simulink model "OFDM_QPSK_Rayleigh_Channel"  (Simulink 7.9)
settings: Solver=FixedStepDiscrete  StartTime=0.0  StopTime=1000  RelTol=1e-3
PreLoadFcn:
  | bitRate = 500000;
  | bitsPerFrame = 200;
  | maxDopplerShift = 200;
  | delayVector = [0:3]*(4e-6);
  | gainVector = [0:3]*(-3);
  | LOSDopplerShift = 100;
  | KFactor = 10;
undefined symbols (not defined in the file or in its folder): figposition, Fs, get, sided, Two
libraries: dspxfrm3 x4, commchan3 x3, commsink2 x2, dspsnks4 x1, dspstat3 x1, commrandsrc2 x1, commdigbbndam3 x1
Description:
  | Multipath Fading Channel
  | 
  | To learn about this model, click <a href="matlab: showdemo multipathfading_demo;">here</a>.
CloseFcn:
  | clear bitRate
  | clear bitsPerFrame
  | clear maxDopplerShift
  | clear delayVector
  | clear gainVector
  | clear LOSDopplerShift
  | clear KFactor
settings Model: Creator=The MathWorks Inc.  LastModifiedBy=leixia  ExtModeAutoUpdateStatusClock=off  BufferReuse=off
settings DataIOCC: LimitDataPoints=off  SaveOutput=off  SignalLogging=off  SaveTime=off  SignalLoggingName=multipathSigsOut
settings OptimizationCC: BooleanDataType=off  InlineInvariantSignals=on  OptimizeBlockIOStorage=off  BufferReuse=off  ExpressionFolding=off  LocalBlockOutputs=off  InitFltsAndDblsToZero=on  BufferReusableBoundary=off
settings DebuggingCC: SaveWithParameterizedLinksMsg=none  CheckExecutionContextPreStartOutputMsg=on  CheckExecutionContextRuntimeOutputMsg=on  SignalResolutionControl=TryResolveAllWithWarning  SolverPrmCheckMsg=none  InheritedTsInSrcMsg=none  MultiTaskDSMMsg=warning  MultiTaskCondExecSysMsg=none  SigSpecEnsureSampleTimeMsg=none  FcnCallInpInsideContextMsg=Use local settings  BusObjectLabelMismatch=none  StrictBusMsg=None
settings HardwareCC: TargetUnknown=on
settings ModelReferenceCC: UpdateModelReferenceTargets=IfOutOfDate
settings RTWCC: IncludeERTFirstTime=on
settings GRTTargetCC: TargetFcnLib=ansi_tfl_tmw.mat  CombineOutputUpdateFcns=off  GRTInterface=on

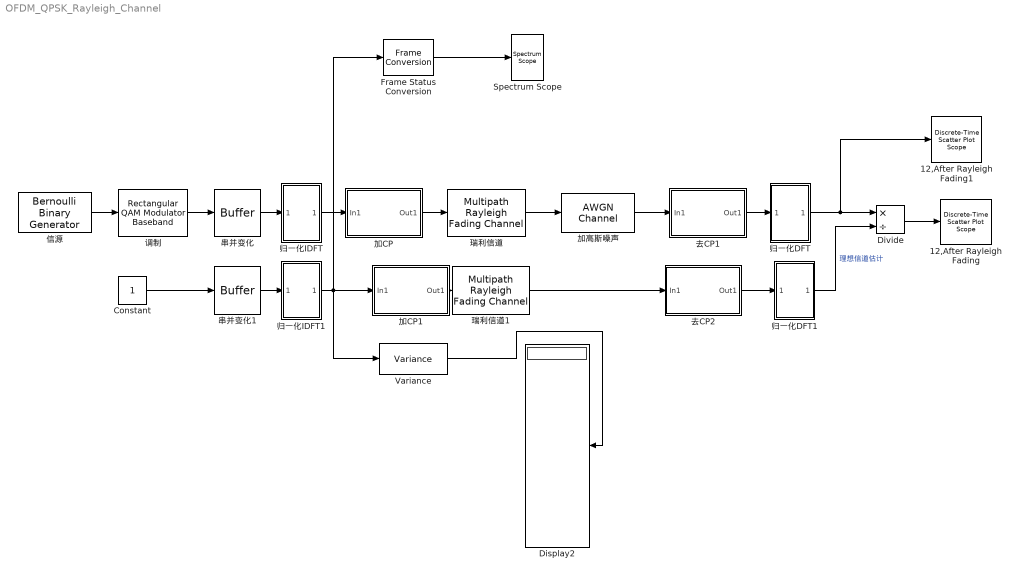
== system OFDM_QPSK_Rayleigh_Channel ==
  12,After Rayleigh Fading : commsink2/Discrete-Time Scatter Plot Scope  Tag=ScatterPlot  sampPerSymb=1  offsetEye=0  numTraces=100  numNewFrames=8  LineMarkers=.  LineColors=b  fading=on  render=on  AxisGrid=on  xMin=-1.2  xMax=1.2  yMin=-1.2  yMax=1.2  inphaseLabel=In-phase Amplitude  quadratureLabel=Quadrature Amplitude  openScopeAtSimStart=off  FrameNumber=off  FigPos=figposition([1 40 25 40])  figTitle=Received signal after Rayleigh fading  numLinesMax=8  block_type_=scatter
  12,After Rayleigh Fading1 : commsink2/Discrete-Time Scatter Plot Scope  Tag=ScatterPlot  sampPerSymb=1  offsetEye=0  numTraces=100  numNewFrames=8  LineMarkers=.  LineColors=b  fading=on  render=on  AxisGrid=on  xMin=-1.2  xMax=1.2  yMin=-1.2  yMax=1.2  inphaseLabel=In-phase Amplitude  quadratureLabel=Quadrature Amplitude  openScopeAtSimStart=off  FrameNumber=off  FigPos=figposition([1 40 25 40])  figTitle=Received signal after Rayleigh fading  numLinesMax=8  block_type_=scatter
  Constant : Constant  VectorParams1D=off  SampleTime=1/500000*2  FramePeriod=256
  Display2 : Display
  Divide : Product  Inputs=*/
  Frame Status Conversion : FrameConversion
  Spectrum Scope : dspsnks4/Spectrum Scope  ScopeProperties=on  Domain=Frequency  HorizSpan=1  UseBuffer=off  BufferSize=272  Overlap=0  TreatMby1Signals=One channel  inpFftLenInherit=off  FFTlength=272  numAvg=1  DisplayProperties=off  AxisGrid=on  Memory=off  FrameNumber=on  AxisLegend=off  AxisZoom=off  OpenScopeAtSimStart=on  OpenScopeImmediately=off  FigPos=get(0,'defaultfigureposition')  AxisProperties=off  XUnits=Hertz  XRange=Two-sided ((-Fs/2...Fs/2])  XDisplay=0  InheritXIncr=on  XIncr=1.0  XLabel=Samples  XLimit=Auto  YUnits=dBW/Hertz  XMax=1  XMin=0  YLabel=Magnitude-squared, dB  LineProperties=off  wintypeSpecScope=Hann  RsSpecScope=50  betaSpecScope=5  winsampSpecScope=Periodic  XAxisParamsVer=6.9  isFrameUpgraded=on
      settings: YMin=-10  YMax=10
  Variance : dspstat3/Variance  run=on  reset_popup=None  InputProcessing=Columns as channels (frame based)  directionMode=Each column  dimension=1  treatSBRowAsCol=on  roiEnable=off  roiType=Rectangles  roiPortion=Entire ROI  roiOutput=Individual statistics for each ROI  roiFlag=off  roundingMode=Floor  overflowMode=off
  串并变化 : Buffer  N=256  TreatMby1Signals=One channel
  串并变化1 : Buffer  N=256  TreatMby1Signals=One channel
  信源 : commrandsrc2/Bernoulli Binary Generator  P=0.5  seed=61  Ts=1/500000  frameBased=on  sampPerFrame=2  orient=off  outDataType=double
  加CP : Subsystem
  加CP1 : Subsystem
  加高斯噪声 : commchan3/AWGN Channel  InputProcessing=Inherited (this choice will be removed - see release notes)  seed=67  noiseMode="Signal to noise ratio  (SNR)"  EbNodB=10  EsNodB=15  SNRdB=200  bitsPerSym=1  Ps=1  Tsym=1e-6  variance=1
  去CP1 : Subsystem
  去CP2 : Subsystem
  归一化DFT : Subsystem
  归一化DFT1 : Subsystem
  归一化IDFT : Subsystem
  归一化IDFT1 : Subsystem
  瑞利信道 : commchan3/Multipath Rayleigh Fading Channel  maxDopplerShift=0.01  spectrumType=Jakes  sigmaGaussian=1/sqrt(2)  coeffRounded=[1 -1.72 0.785]  freqMinMaxRJakes=[0 1]  freqMinMaxAJakes=[0 1]  sigmaGaussian1=1/sqrt(2)  sigmaGaussian2=1/sqrt(2)  centerFreqGaussian1=0.0  centerFreqGaussian2=0.0  gainGaussian1=0.5  gainGaussian2=0.5  coeffBell=9  dopplerSpectrum=doppler.jakes  pathDelays="[ 0    0.0400 ].*1e-4"  avgPathGaindB="[ 0    -3 ]"  normalizePathGains=on  seed=12345  enableProbe=0  openVisAtStart=off  outPathGains=off  outDelay=off
  瑞利信道1 : commchan3/Multipath Rayleigh Fading Channel  maxDopplerShift=0.01  spectrumType=Jakes  sigmaGaussian=1/sqrt(2)  coeffRounded=[1 -1.72 0.785]  freqMinMaxRJakes=[0 1]  freqMinMaxAJakes=[0 1]  sigmaGaussian1=1/sqrt(2)  sigmaGaussian2=1/sqrt(2)  centerFreqGaussian1=0.0  centerFreqGaussian2=0.0  gainGaussian1=0.5  gainGaussian2=0.5  coeffBell=9  dopplerSpectrum=doppler.jakes  pathDelays="[ 0    0.0400 ].*1e-4"  avgPathGaindB="[ 0    -3 ]"  normalizePathGains=on  seed=12345  enableProbe=0  openVisAtStart=off  outPathGains=off  outDelay=off
  调制 : commdigbbndam3/Rectangular QAM Modulator Baseband  M=4  InType=Bit  Enc=Gray  Mapping=[0,1,2,3]  PowType=Average Power  MinDist=2  AvgPow=1  PeakPow=1  Ph=-pi/2  outDtype=double  outWordLen=16  outUDDataType=sfix(16)  outFracLenMode=Best precision  outFracLen=15
  wires:
  调制/1 -> 串并变化/1
  瑞利信道/1 -> 加高斯噪声/1
  加高斯噪声/1 -> 去CP1/1(In1)
  信源/1 -> 调制/1
  加CP/1(Out1) -> 瑞利信道/1
  归一化IDFT/1(Out1) -> 加CP/1(In1)
  串并变化/1 -> 归一化IDFT/1(In1)
  去CP1/1(Out1) -> 归一化DFT/1(In1)
  去CP2/1(Out1) -> 归一化DFT1/1(In1)
  加CP1/1(Out1) -> 瑞利信道1/1
  Constant/1 -> 串并变化1/1
  串并变化1/1 -> 归一化IDFT1/1(In1)
  瑞利信道1/1 -> 去CP2/1(In1)
  归一化DFT/1(Out1) -> Divide/1, 12,After Rayleigh Fading1/1
  归一化DFT1/1(Out1) -> Divide/2  "理想信道估计"
  Divide/1 -> 12,After Rayleigh Fading/1
  Frame Status Conversion/1 -> Spectrum Scope/1
  归一化IDFT1/1(Out1) -> Frame Status Conversion/1, 加CP1/1(In1), Variance/1
  Variance/1 -> Display2/1

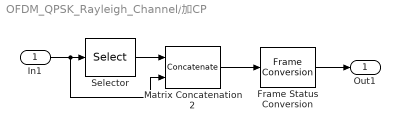
== system OFDM_QPSK_Rayleigh_Channel/加CP ==
  In1 : Inport
  Frame Status Conversion : FrameConversion
  Matrix Concatenation2 : Concatenate
  Selector : Selector  InputPortWidth=256  IndexOptions=Index vector (dialog)  Indices=[256-16+1:1:256]  OutputSizes=1
  Out1 : Outport
  wires:
  Selector/1 -> Matrix Concatenation2/1
  In1/1 -> Matrix Concatenation2/2, Selector/1
  Matrix Concatenation2/1 -> Frame Status Conversion/1
  Frame Status Conversion/1 -> Out1/1

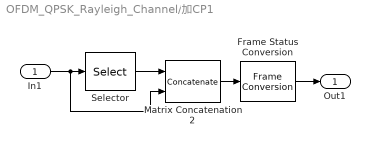
== system OFDM_QPSK_Rayleigh_Channel/加CP1 ==
  In1 : Inport
  Frame Status Conversion : FrameConversion
  Matrix Concatenation2 : Concatenate
  Selector : Selector  InputPortWidth=256  IndexOptions=Index vector (dialog)  Indices=[256-16+1:1:256]  OutputSizes=1
  Out1 : Outport
  wires:
  Frame Status Conversion/1 -> Out1/1
  Matrix Concatenation2/1 -> Frame Status Conversion/1
  In1/1 -> Selector/1, Matrix Concatenation2/2
  Selector/1 -> Matrix Concatenation2/1

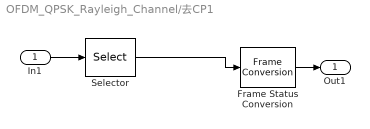
== system OFDM_QPSK_Rayleigh_Channel/去CP1 ==
  In1 : Inport
  Frame Status Conversion : FrameConversion
  Selector : Selector  InputPortWidth=256+16  IndexOptions=Index vector (dialog)  Indices=[16+1:1:256+16]  OutputSizes=1
  Out1 : Outport
  wires:
  Frame Status Conversion/1 -> Out1/1
  In1/1 -> Selector/1
  Selector/1 -> Frame Status Conversion/1

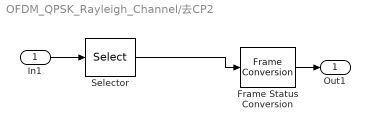
== system OFDM_QPSK_Rayleigh_Channel/去CP2 ==
  In1 : Inport
  Frame Status Conversion : FrameConversion
  Selector : Selector  InputPortWidth=256+16  IndexOptions=Index vector (dialog)  Indices=[16+1:1:256+16]  OutputSizes=1
  Out1 : Outport
  wires:
  Selector/1 -> Frame Status Conversion/1
  In1/1 -> Selector/1
  Frame Status Conversion/1 -> Out1/1

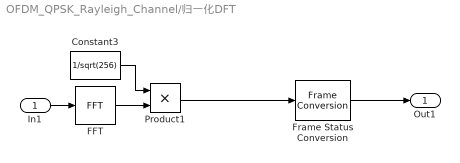
== system OFDM_QPSK_Rayleigh_Channel/归一化DFT ==
  In1 : Inport
  Constant3 : Constant  Value=1/sqrt(256)
  FFT : dspxfrm3/FFT  CompMethod=Table lookup  TableOpt=NEW  TableOptActive=Speed  BitRevOrder=off  InheritFFTLength=on  FFTLength=64  RowConvenienceOn=on  FFTImplementation=Auto  SkipNorm=off  firstCoeffDataTypeStr=Inherit: Same word length as input  firstCoeffLastDataTypeStr=Inherit: Same word length as input  outputMin=[]  outputMax=[]  roundingMode=Floor  overflowMode=off
  Frame Status Conversion : FrameConversion
  Product1 : Product  SaturateOnIntegerOverflow=on  InputSameDT=on  OutDataTypeStr=Inherit: Same as first input
  Out1 : Outport
  wires:
  In1/1 -> FFT/1
  Product1/1 -> Frame Status Conversion/1
  FFT/1 -> Product1/2
  Constant3/1 -> Product1/1
  Frame Status Conversion/1 -> Out1/1

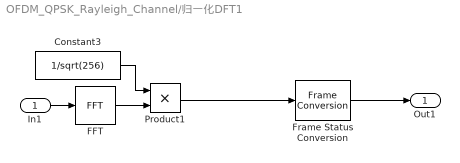
== system OFDM_QPSK_Rayleigh_Channel/归一化DFT1 ==
  In1 : Inport
  Constant3 : Constant  Value=1/sqrt(256)
  FFT : dspxfrm3/FFT  CompMethod=Table lookup  TableOpt=NEW  TableOptActive=Speed  BitRevOrder=off  InheritFFTLength=on  FFTLength=64  RowConvenienceOn=on  FFTImplementation=Auto  SkipNorm=off  firstCoeffDataTypeStr=Inherit: Same word length as input  firstCoeffLastDataTypeStr=Inherit: Same word length as input  outputMin=[]  outputMax=[]  roundingMode=Floor  overflowMode=off
  Frame Status Conversion : FrameConversion
  Product1 : Product  SaturateOnIntegerOverflow=on  InputSameDT=on  OutDataTypeStr=Inherit: Same as first input
  Out1 : Outport
  wires:
  Frame Status Conversion/1 -> Out1/1
  Constant3/1 -> Product1/1
  FFT/1 -> Product1/2
  Product1/1 -> Frame Status Conversion/1
  In1/1 -> FFT/1

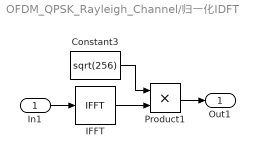
== system OFDM_QPSK_Rayleigh_Channel/归一化IDFT ==
  In1 : Inport
  Constant3 : Constant  Value=sqrt(256)
  IFFT : dspxfrm3/IFFT  CompMethod=Table lookup  TableOpt=NEW  TableOptActive=Speed  BitRevOrder=off  cs_in=off  SkipNorm=on  InheritFFTLength=on  FFTLength=64  mode=Complex  outSamplingMode=Sample based  RowConvenienceOn=on  FFTImplementation=Auto  firstCoeffDataTypeStr=Inherit: Same word length as input  firstCoeffLastDataTypeStr=Inherit: Same word length as input  outputMin=[]  outputMax=[]  roundingMode=Floor  overflowMode=off
  Product1 : Product  SaturateOnIntegerOverflow=on  InputSameDT=on  OutDataTypeStr=Inherit: Same as first input
  Out1 : Outport
  wires:
  Constant3/1 -> Product1/1
  IFFT/1 -> Product1/2
  Product1/1 -> Out1/1
  In1/1 -> IFFT/1

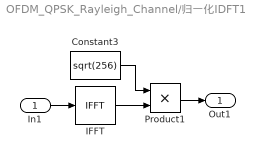
== system OFDM_QPSK_Rayleigh_Channel/归一化IDFT1 ==
  In1 : Inport
  Constant3 : Constant  Value=sqrt(256)
  IFFT : dspxfrm3/IFFT  CompMethod=Table lookup  TableOpt=NEW  TableOptActive=Speed  BitRevOrder=off  cs_in=off  SkipNorm=on  InheritFFTLength=on  FFTLength=64  mode=Complex  outSamplingMode=Sample based  RowConvenienceOn=on  FFTImplementation=Auto  firstCoeffDataTypeStr=Inherit: Same word length as input  firstCoeffLastDataTypeStr=Inherit: Same word length as input  outputMin=[]  outputMax=[]  roundingMode=Floor  overflowMode=off
  Product1 : Product  SaturateOnIntegerOverflow=on  InputSameDT=on  OutDataTypeStr=Inherit: Same as first input
  Out1 : Outport
  wires:
  In1/1 -> IFFT/1
  Product1/1 -> Out1/1
  IFFT/1 -> Product1/2
  Constant3/1 -> Product1/1
